simulink subsystem "mmc_hb_arm"  (R2026a)
settings: Solver=VariableStepAuto
settings Model: Creator=zheng  LastModifiedBy=zheng

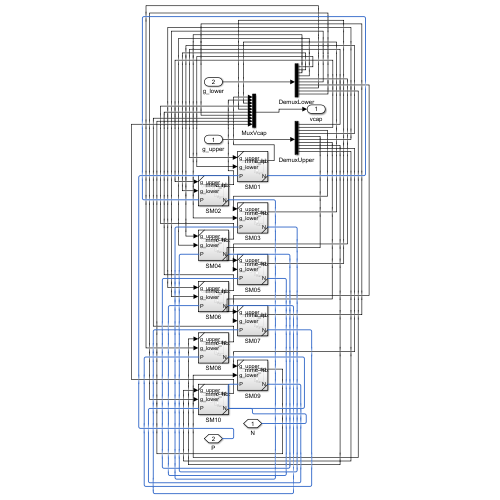
[thumbnail: Simulink's stored preview of the top-level diagram]
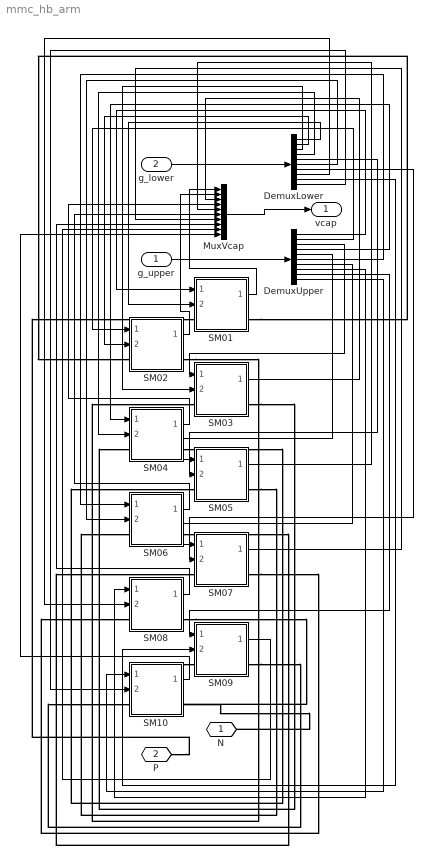
== system mmc_hb_arm ==
  g_upper : Inport
  g_lower : Inport  Port=2
  DemuxLower : Demux  Outputs=10
  DemuxUpper : Demux  Outputs=10
  MuxVcap : Mux  Inputs=10
  SM01 : Subsystem  ReferencedSubsystem=mmc_hb_submodule
  SM02 : Subsystem  ReferencedSubsystem=mmc_hb_submodule
  SM03 : Subsystem  ReferencedSubsystem=mmc_hb_submodule
  SM04 : Subsystem  ReferencedSubsystem=mmc_hb_submodule
  SM05 : Subsystem  ReferencedSubsystem=mmc_hb_submodule
  SM06 : Subsystem  ReferencedSubsystem=mmc_hb_submodule
  SM07 : Subsystem  ReferencedSubsystem=mmc_hb_submodule
  SM08 : Subsystem  ReferencedSubsystem=mmc_hb_submodule
  SM09 : Subsystem  ReferencedSubsystem=mmc_hb_submodule
  SM10 : Subsystem  ReferencedSubsystem=mmc_hb_submodule
  N : PMIOPort  Side=Right  ConnectionType=Connection: foundation.electrical.electrical
  P : PMIOPort  Port=2  Side=Left  ConnectionType=Connection: foundation.electrical.electrical
  vcap : Outport
  wires:
  g_upper/1 -> DemuxUpper/1
  g_lower/1 -> DemuxLower/1
  MuxVcap/1 -> vcap/1
  DemuxUpper/1 -> SM01/1
  DemuxLower/1 -> SM01/2
  SM01/1 -> MuxVcap/1
  DemuxUpper/2 -> SM02/1
  DemuxLower/2 -> SM02/2
  SM02/1 -> MuxVcap/2
  DemuxUpper/3 -> SM03/1
  DemuxLower/3 -> SM03/2
  SM03/1 -> MuxVcap/3
  DemuxUpper/4 -> SM04/1
  DemuxLower/4 -> SM04/2
  SM04/1 -> MuxVcap/4
  DemuxUpper/5 -> SM05/1
  DemuxLower/5 -> SM05/2
  SM05/1 -> MuxVcap/5
  DemuxUpper/6 -> SM06/1
  DemuxLower/6 -> SM06/2
  SM06/1 -> MuxVcap/6
  DemuxUpper/7 -> SM07/1
  DemuxLower/7 -> SM07/2
  SM07/1 -> MuxVcap/7
  DemuxUpper/8 -> SM08/1
  DemuxLower/8 -> SM08/2
  SM08/1 -> MuxVcap/8
  DemuxUpper/9 -> SM09/1
  DemuxLower/9 -> SM09/2
  SM09/1 -> MuxVcap/9
  DemuxUpper/10 -> SM10/1
  DemuxLower/10 -> SM10/2
  SM10/1 -> MuxVcap/10
  connections:
  P/RConn1 -- SM01/LConn1
  SM01/RConn1 -- SM02/LConn1
  SM02/RConn1 -- SM03/LConn1
  SM03/RConn1 -- SM04/LConn1
  SM04/RConn1 -- SM05/LConn1
  SM05/RConn1 -- SM06/LConn1
  SM06/RConn1 -- SM07/LConn1
  SM07/RConn1 -- SM08/LConn1
  SM08/RConn1 -- SM09/LConn1
  SM09/RConn1 -- SM10/LConn1
  SM10/RConn1 -- N/RConn1
